simulink model "VEHICLE_DYN_TRAIN"  (R2019b)
settings: Solver=ode4  StartTime=0.0  StopTime=150  FixedStep=0.01  RelTol=1e-3
model workspace (MAT data in the model file):
  ACCEL = [0 0.000975932898663 -0.0414538855996 0.0440661905922 -0.0484817487001 0.0392964510644 -0.0693895143615 0.0261566921783 -0.0586295561215 0.0249771458914 -0.0595081132089 0.0233316013131 ... (544 elements, 17x32)]
  A_mc = 0.000491
  CMD_BR = [0 0 0 0 0 0 0 0 0 0 0 0 ... (15001 elements, 15001x1)]
  CMD_MODE = [1 1 1 1 1 1 1 1 1 1 1 1 ... (15001 elements, 15001x1)]
  CMD_ST = [0 0 0 0 0 0 0 0 0 0 0 0 ... (15001 elements, 15001x1)]
  CMD_T = [0 0.01 0.02 0.03 0.04 0.05 0.06 0.07 0.08 0.09 0.1 0.11 ... (2001 elements, 1x2001)]
  CMD_TH = [0 0 0 0 0 0 0 0 0 0 0 0 ... (15001 elements, 15001x1)]
  CMD_TM = [0 0.01 0.02 0.03 0.04 0.05 0.06 0.07 0.08 0.09 0.1 0.11 ... (15001 elements, 15001x1)]
  CMD_U = [10 10 10 10 10 10 10 10 10 10 10 10 ... (2001 elements, 1x2001)]
  CMD_UX = [0.1 0.1 0.1 0.1 0.1 0.1 0.1 0.1 0.1 0.1 0.1 0.1 ... (15001 elements, 15001x1)]
  COMMAND = [0 0 0 0 0 0 0 0 0 0 0 0 ... (102 elements, 17x6)]
  C_q = 1.4e-06
  DATA_HMMWV : object (value not decoded)
  DATA_VESIM_CC_BRAKE : object (value not decoded)
  FORCE = [0 -4628.45620853 2357.84853747 -1841.82564621 -1727.75397473 1695.19792057 -1263.06335256 1524.31841051 -1649.98396845 -1537.1025145 -1335.96213703 1639.88309903 ... (493 elements, 17x29)]
  F_cf = 80
  F_cs = 138
  F_z = -50097.6
  Gain_v = 70
  J_wheel = 32
  K_vb = 1500
  Kp_rpm = 2.7013
  Kp_v = 30
  L3 = 10
  MIN_TH = 0
  M_sprung = 4672
  M_unsprung = 220
  M_unsprung_front = 220
  M_vehicle = 5112
  N2 = 0
  N3 = 0.01
  P = 36
  P_0 = 10670
  P_gain = 0.0006
  R_wheel = 0.4412
  SLIP = [0 -0.5 0.5 -0.5 -0.5 0.5 -0.5 0.5 -0.5 -0.5 -0.5 0.5 ... (136 elements, 17x8)]
  STATE = [0 4.33747954961e-06 -0.000147430460781 -3.72129119222e-05 -0.000284189368187 -0.000207128204422 -0.00055150808757 -0.000594561033148 -0.000967775941564 -0.00103412952076 -0.00143215770154 -0.00152470872631 ... (544 elements, 17x32)]
  STATES_INIT = [0 0 0.9902452 0 0 1.57079632679 0.01 0 0 0 0 0 ... (32 elements, 1x32)]
  SUSP = [0 -0.00875795294893 -0.00878173856984 -0.00830852863719 -0.00873591176348 -0.00870428588158 -0.00751721170558 -0.00851904716693 -0.00789923296531 -0.00838039895253 -0.00756270047902 -0.00866403364289 ... (612 elements, 17x36)]
  S_o = 3
  T2_r = 4
  TIRE = [0 0.0910654620457 -0.0936729683319 0.0717372732987 0.0513932148365 -0.0365035701266 -0.00739813929507 -0.0045484168787 0.0723881675257 0.0296400174207 -0.0169805208571 0.0207214713062 ... (408 elements, 17x24)]
  TIRELIFTOFF = [0 0 0 0 0 0 0 0 0 0 0 0 ... (17 elements, 17x1)]
  T_LENGTH = 2001
  T_STEP = 0.01
  T_STOP = 12.82
  T_TOTAL = 20
  Ti_rpm = 0.6464
  Ti_v = 2.5
  Tstop = [150 150 150 150 150 150 150 150 150 150 150 150 ... (15001 elements, 15001x1)]
  Tt_rpm = 0.0808
  Tt_v = 0.3125
  U_INIT = 0.01
  b = 170
  brake_Pw = [-3.96235801772 -3.96238075942 -0.895107722214 -0.895547395081 35.9159438465 72.7273668629 152.485661058 244.514654481 330.408495385 364.152342142 462.316700341 535.939857177 ... (40 elements, 40x1)]
  brake_V = [-1.14468402636e-08 6.09303685082e-09 2.9257815427e-07 6.31682445149e-07 8.18779962309e-07 1.05849711081e-06 1.41515318379e-06 1.67826507702e-06 1.8361367918e-06 2.02323385108e-06 2.22788040303e-06 2.46760304614e-06 ... (40 elements, 40x1)]
  diff_efficiency = 0.94
  diff_wRatio = 6.052
  diff_w_ratio = 3.56
  end_time = 140
  engine_inertia = 0.53
  fmin_mg = [42.75 43.31 51.6 64.3 73.65 71.1 72.7 72.36]
  fmin_mg_na = [42.79 42.79 42.79 42.79 42.79 42.79 42.79 42.79]
  g = -9.8
  g_motor_eff = 1
  gr_motor = 0
  i = 5
  mdot_fuel = [5e-06 1e-05 2e-05 3e-05 4e-05 5e-05 6e-05 7e-05 8e-05]
  ms2mph = 2.23694
  n_tire = 4
  no_cyl = 8
  num_points = 14000
  num_points_fast = 140000
  rpm0 = 83.7758040957
  rpm0_c = 1000
  rpm2rads = 0.10471975512
  rpm_e = [50 800 1000 1500 2000 2500 3000 3300]
  rpm_engine = [700 800 1000 1500 2000 2500 3000 3300]
  rpm_hi_idle = 3400
  rpm_idle = 750
  rpm_max_c = 3200
  rpm_rated = 3200
  start_time = 0
  time_step = 0.01
  time_step_fast = 0.001
  torque_engine = [9.767 15.303 12.411 -4.524 -12.214 -35.77 -70 -75.889 75.383 80.318 76.501 61.314 ... (72 elements, 8x9)]
  tout = [0 0.01 0.02 0.03 0.04 0.05 0.06 0.07 0.08 0.09 0.1 0.11 ... (17 elements, 17x1)]
  trq_scale = 0.46
values from neighbouring files (symbols this model uses):
  B = Ref(i:i+2,2)    [Calc_vref.m]    (also in Parameter_load.m = 0.1; VEHICLE_DYN_TRAIN_INIT.m = 0.25)
  Error_now = Error_now_array(end)    [RUN_SIMULATION_SHARED_NEW_POWERTRAIN.m]    (also in VEHICLE_DYN_TRAIN_INIT.m = 0)
  J = 0.075    [VEHICLE_DYN_TRAIN_INIT.m]
  K = 0.075    [VEHICLE_DYN_TRAIN_INIT.m]
  pid2tau_gain = 2.5    [VEHICLE_DYN_TRAIN_INIT.m]
  st_a_in = st_sc_out(end)    [RUN_SIMULATION_SHARED_NEW_POWERTRAIN.m]    (also in VEHICLE_DYN_TRAIN_INIT.m = 0)
  tau_a_in = tau_a_out(end)    [RUN_SIMULATION_SHARED_NEW_POWERTRAIN.m]    (also in VEHICLE_DYN_TRAIN_INIT.m = 0)
undefined symbols (not defined in the file or in its folder): adaptive_flag, autonomy_human_contain_gain, Bias_Distance, dt, error_lookuptable, human_autonomy_agreement_threshold, human_contain_min, human_response_dead_zone, human_torque_max, J_cal, kp_sc, model_lookuptable, Standard_Devices, steering_stable_threshold, UDP_Protocol, vdes, Xobs, Yobs
libraries: simulink x16, sldrtlib x3, dspstat3 x3, vrlib x2
(part 3 of 4)

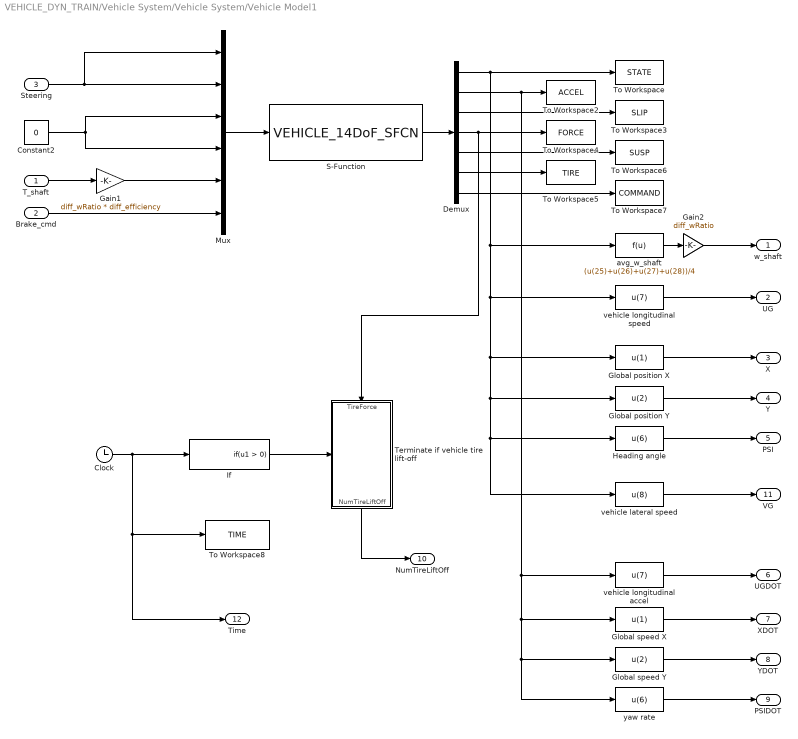
== system VEHICLE_DYN_TRAIN/Vehicle System/Vehicle System/Vehicle Model1 ==
  T_shaft : Inport
  Brake_cmd : Inport  Port=2
  Steering : Inport  Port=3
  Clock : Clock
  Constant2 : Constant  Value=0
  Demux : Demux  Outputs=[32,32,8,29,36,24,6]
  Gain1 : Gain  Gain=diff_wRatio * diff_efficiency
  Gain2 : Gain  Gain=diff_wRatio
  Global position X : Fcn  Expr=u(1)
  Global position Y : Fcn  Expr=u(2)
  Global speed X : Fcn  Expr=u(1)
  Global speed Y : Fcn  Expr=u(2)
  Heading angle : Fcn  Expr=u(6)
  If : If  ShowElse=off
  Mux : Mux  Inputs=6
  S-Function : S-Function  FunctionName=VEHICLE_14DoF_SFCN  SFunctionDeploymentMode=off  EnableBusSupport=off
  Terminate if vehicle tire lift-off : Subsystem  TreatAsAtomicUnit=on
  To Workspace : ToWorkspace  VariableName=STATE  SampleTime=-1
  To Workspace2 : ToWorkspace  VariableName=ACCEL  SampleTime=-1
  To Workspace3 : ToWorkspace  VariableName=SLIP  SampleTime=-1
  To Workspace4 : ToWorkspace  VariableName=FORCE  SampleTime=-1
  To Workspace5 : ToWorkspace  VariableName=TIRE  SampleTime=-1
  To Workspace6 : ToWorkspace  VariableName=SUSP  SampleTime=-1
  To Workspace7 : ToWorkspace  VariableName=COMMAND  SampleTime=-1
  To Workspace8 : ToWorkspace  VariableName=TIME  SampleTime=-1
  avg_w_shaft : Fcn  Expr=(u(25)+u(26)+u(27)+u(28))/4
  vehicle lateral speed : Fcn  Expr=u(8)
  vehicle longitudinal accel : Fcn  Expr=u(7)
  vehicle longitudinal speed : Fcn  Expr=u(7)
  yaw rate : Fcn  Expr=u(6)
  w_shaft : Outport  VectorParamsAs1DForOutWhenUnconnected=off
  UG : Outport  Port=2  VectorParamsAs1DForOutWhenUnconnected=off
  X : Outport  Port=3  VectorParamsAs1DForOutWhenUnconnected=off
  Y : Outport  Port=4  VectorParamsAs1DForOutWhenUnconnected=off
  PSI : Outport  Port=5  VectorParamsAs1DForOutWhenUnconnected=off
  UGDOT : Outport  Port=6  VectorParamsAs1DForOutWhenUnconnected=off
  XDOT : Outport  Port=7  VectorParamsAs1DForOutWhenUnconnected=off
  YDOT : Outport  Port=8  VectorParamsAs1DForOutWhenUnconnected=off
  PSIDOT : Outport  Port=9  VectorParamsAs1DForOutWhenUnconnected=off
  NumTireLiftOff : Outport  Port=10  VectorParamsAs1DForOutWhenUnconnected=off
  VG : Outport  Port=11  VectorParamsAs1DForOutWhenUnconnected=off
  Time : Outport  Port=12  VectorParamsAs1DForOutWhenUnconnected=off
  wires:
  Demux/3 -> To Workspace3/1
  Constant2/1 -> Mux/3, Mux/4
  Demux/5 -> To Workspace6/1
  Steering/1 -> Mux/1, Mux/2
  avg_w_shaft/1 -> Gain2/1
  T_shaft/1 -> Gain1/1
  Demux/7 -> To Workspace7/1
  Demux/1 -> To Workspace/1, vehicle lateral speed/1, Heading angle/1, Global position Y/1, Global position X/1, vehicle longitudinal speed/1, avg_w_shaft/1
  Mux/1 -> S-Function/1
  vehicle longitudinal speed/1 -> UG/1
  Demux/6 -> To Workspace5/1
  Brake_cmd/1 -> Mux/6
  S-Function/1 -> Demux/1
  Heading angle/1 -> PSI/1
  Gain2/1 -> w_shaft/1
  Gain1/1 -> Mux/5
  Global position X/1 -> X/1
  Global position Y/1 -> Y/1
  yaw rate/1 -> PSIDOT/1
  Demux/2 -> vehicle longitudinal accel/1, Global speed X/1, Global speed Y/1, yaw rate/1, To Workspace2/1
  vehicle longitudinal accel/1 -> UGDOT/1
  Global speed X/1 -> XDOT/1
  Global speed Y/1 -> YDOT/1
  Demux/4 -> Terminate if vehicle tire lift-off/1(TireForce), To Workspace4/1
  If/1 -> Terminate if vehicle tire lift-off/Action
  Terminate if vehicle tire lift-off/1(NumTireLiftOff) -> NumTireLiftOff/1
  vehicle lateral speed/1 -> VG/1
  Clock/1 -> Time/1, To Workspace8/1, If/1

== system VEHICLE_DYN_TRAIN/Autonomy/Subsystem/Distance Indicator/Subsystem1 ==
  XG : Inport
  YG : Inport  Port=2
  X_init : Inport  Port=3
  Constant : Constant  Value=0.01
  MATLAB Function : MATLAB Function  TreatAsAtomicUnit=on
  DisInfo : Outport  VectorParamsAs1DForOutWhenUnconnected=off
  X_init_update : Outport  Port=2  VectorParamsAs1DForOutWhenUnconnected=off
  wires:
  X_init/1 -> MATLAB Function/3(Xinit)
  YG/1 -> MATLAB Function/2(Yv)
  XG/1 -> MATLAB Function/1(Xv)
  Constant/1 -> MATLAB Function/4(alpha)
  MATLAB Function/1(Xinit_final) -> X_init_update/1
  MATLAB Function/2(distance) -> DisInfo/1

== system VEHICLE_DYN_TRAIN/Vehicle System/Vehicle System/Powertrain1/DIESEL ENGINE ==
  note: RPM
  note: If you are using MATLAB 6 or earlier,
      | double-click on this look-up table and
      | make sure the "Table data" entry is torque_engine
  engine speed : Inport
  driver  demand : Inport  Port=2
  Engine Map : Lookup2D  RowIndex=rpm_engine  ColumnIndex=mdot_fuel*1e3  Table=torque_engine  SaturateOnIntegerOverflow=on  InputSameDT=on
  Fuel controller/ Governor : Subsystem
  Gain : Gain  Gain=trq_scale  SaturateOnIntegerOverflow=on  OutDataTypeStr=Inherit: Same as input  ParamDataTypeStr=Inherit: Same as input
  Idle Controller : Subsystem
  Mux2 : Mux  Inputs=2
  To File1 : ToFile  Filename=Powertrain_data/engine_NO.mat  MatrixName=engine_out
  radpersec2rpm : Gain  Gain=1/rpm2rads
  engine torque : Outport  VectorParamsAs1DForOutWhenUnconnected=off
  wires:
  radpersec2rpm/1 -> Engine Map/1, Fuel controller/ Governor/2(rpm), Idle Controller/1(engine speed), Mux2/2
  engine speed/1 -> radpersec2rpm/1
  Fuel controller/ Governor/1(mdot_fuel) -> Engine Map/2
  Idle Controller/1(rack) -> Fuel controller/ Governor/1(Rack)
  Gain/1 -> engine torque/1, Mux2/1
  Mux2/1 -> To File1/1
  driver  demand/1 -> Idle Controller/2(driver command)
  Engine Map/1 -> Gain/1

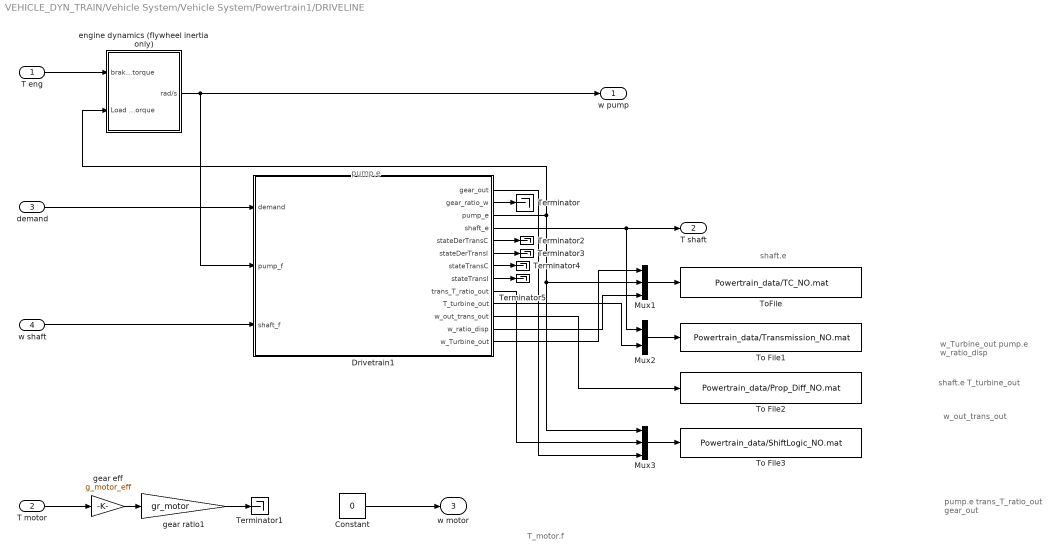
== system VEHICLE_DYN_TRAIN/Vehicle System/Vehicle System/Powertrain1/DRIVELINE ==
  note: pump.e
  note: shaft.e
  note: T_motor.f
  note: w_Turbine_out
      | pump.e
      | w_ratio_disp
  note: shaft.e
      | T_turbine_out
  note: w_out_trans_out
  note: pump.e
      | trans_T_ratio_out
      | gear_out
  "T eng " : Inport
  T motor : Inport  Port=2
  demand : Inport  Port=3
  w shaft : Inport  Port=4
  Constant : Constant  Value=0
  Drivetrain1 : Subsystem  mask(20-sim 4.1 S-Function block){}
      mask help:
      | This block is generated by the 20-sim ANSI-C Code Generator.
      |
      | * look under the mask to get information on the ports
      | * press Help for more detailed information
      | * the parameters of this block are:
      mask Help:
      | This block is generated by the 20-sim ANSI-C Code Generator<br>
      | The block parameters are:<br><blockquote></blockquote>
      | Generated at:<br>
      | <blockquote><b>date:  </b>November 7, 2011<br>
      | <b>time:  </b>6:10:49 pm<br></blockquote>
      | From the following 20-sim model:<br>
      | <blockquote><b>submodel:  </b>Drivetrain<br>
      | <b>model:  </b>model-based internet integration - original drivetrain params<br>
      | <b>file:  </b>C:\Users\Tulga Ersal\Documents\U of M\Post Doc\Projects\Long-haul HIL integration\20-sim\integration models for 20Sim 4.0.1.5 and up\model-based internet integration - original drivetrain params.emx<br>
      | <b>experiment:  </b>C:\Users\Tulga Ersal\Documents\U of M\Post Doc\Projects\Long-haul HIL integration\20-sim\integration models for 20Sim 4.0.1.5 and up\model-based internet integration - original drivetrain params.emx<br></blockquote>
      | Using the following 20-sim license:<br>
      | <blockquote><b>user:  </b>The University of Michigan<br>
      | <b>from:  </b>Student License<br>
      | <b>build: </b>4.1.0.4<br></blockquote>
      mask Display: disp('Drivetrain')
  Mux1 : Mux  Inputs=3
  Mux2 : Mux  Inputs=2
  Mux3 : Mux  Inputs=3
  Terminator{,1..5} (6 alike) : Terminator
  To File1 : ToFile  Filename=Powertrain_data/Transmission_NO.mat  MatrixName=Transmission_out
  To File2 : ToFile  Filename=Powertrain_data/Prop_Diff_NO.mat  MatrixName=Prop_Diff_out
  To File3 : ToFile  Filename=Powertrain_data/ShiftLogic_NO.mat  MatrixName=ShiftLogic_out
  ToFile : ToFile  Filename=Powertrain_data/TC_NO.mat  MatrixName=TC_out
  engine dynamics (flywheel inertia only) : Subsystem
  gear ratio1 : Gain  Gain=gr_motor  SaturateOnIntegerOverflow=on  OutDataTypeStr=Inherit: Same as input  ParamDataTypeStr=Inherit: Same as input
  gear eff : Gain  Gain=g_motor_eff  SaturateOnIntegerOverflow=on  OutDataTypeStr=Inherit: Same as input  ParamDataTypeStr=Inherit: Same as input
  w pump : Outport  InitialOutput=0  VectorParamsAs1DForOutWhenUnconnected=off
  T shaft : Outport  Port=2  InitialOutput=0  VectorParamsAs1DForOutWhenUnconnected=off
  w motor : Outport  Port=3  InitialOutput=0  VectorParamsAs1DForOutWhenUnconnected=off
  wires:
  "T eng "/1 -> engine dynamics (flywheel inertia only)/1(brake torque)
  engine dynamics (flywheel inertia only)/1(rad/s) -> Drivetrain1/2(pump_f), w pump/1
  demand/1 -> Drivetrain1/1(demand)
  w shaft/1 -> Drivetrain1/3(shaft_f)
  T motor/1 -> gear eff/1
  gear eff/1 -> gear ratio1/1
  Constant/1 -> w motor/1
  Mux1/1 -> ToFile/1
  Mux2/1 -> To File1/1
  Mux3/1 -> To File3/1
  gear ratio1/1 -> Terminator1/1
  Drivetrain1/4(shaft_e) -> T shaft/1, Mux2/1
  Drivetrain1/3(pump_e) -> Mux3/1, Mux1/2, engine dynamics (flywheel inertia only)/2(Load Torque)
  Drivetrain1/13(w_Turbine_out) -> Mux1/1
  Drivetrain1/12(w_ratio_disp) -> Mux1/3
  Drivetrain1/10(T_turbine_out) -> Mux2/2
  Drivetrain1/11(w_out_trans_out) -> To File2/1
  Drivetrain1/9(trans_T_ratio_out) -> Mux3/2
  Drivetrain1/1(gear_out) -> Mux3/3
  Drivetrain1/2(gear_ratio_w) -> Terminator/1
  Drivetrain1/5(stateDerTransC) -> Terminator2/1
  Drivetrain1/6(stateDerTransI) -> Terminator3/1
  Drivetrain1/7(stateTransC) -> Terminator4/1
  Drivetrain1/8(stateTransI) -> Terminator5/1

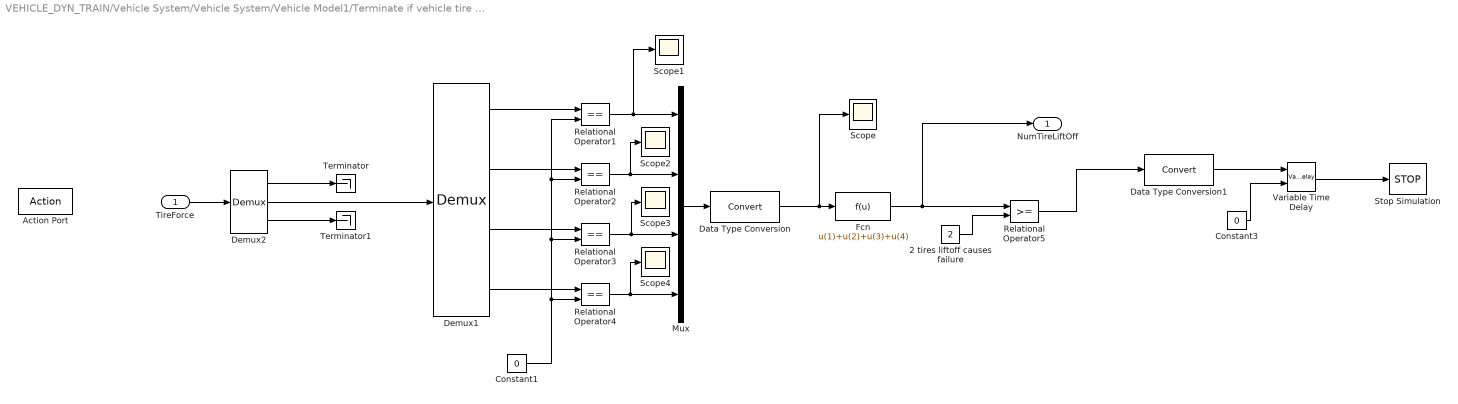
== system VEHICLE_DYN_TRAIN/Vehicle System/Vehicle System/Vehicle Model1/Terminate if vehicle tire lift-off ==
  TireForce : Inport
  Action Port : ActionPort  ActionPortLabel=if(u1 > 0)
  2 tires liftoff causes failure : Constant  Value=2
  Constant1 : Constant  Value=0
  Constant3 : Constant  Value=0
  Data Type Conversion : DataTypeConversion
  Data Type Conversion1 : DataTypeConversion
  Demux1 : Demux
  Demux2 : Demux  Outputs=[8,4,17]
  Fcn : Fcn  Expr=u(1)+u(2)+u(3)+u(4)
  Mux : Mux
  Relational Operator{1..4} (4 alike) : RelationalOperator  Operator===  RndMeth=Nearest  InputSameDT=on
  Relational Operator5 : RelationalOperator  RndMeth=Nearest  InputSameDT=on
  Scope{,1..4} (5 alike) : Scope
  Stop Simulation : Stop
  Terminator : Terminator
  Terminator1 : Terminator
  Variable Time Delay : VariableTransportDelay  MaximumDelay=10  MaximumPoints=10000
  NumTireLiftOff : Outport  InitialOutput=0  VectorParamsAs1DForOutWhenUnconnected=off
  wires:
  Demux2/1 -> Terminator/1
  Demux2/3 -> Terminator1/1
  Demux2/2 -> Demux1/1
  TireForce/1 -> Demux2/1
  Demux1/1 -> Relational Operator1/1
  Demux1/2 -> Relational Operator2/1
  Demux1/3 -> Relational Operator3/1
  Demux1/4 -> Relational Operator4/1
  Relational Operator1/1 -> Scope1/1, Mux/1
  Relational Operator2/1 -> Scope2/1, Mux/2
  Relational Operator3/1 -> Scope3/1, Mux/3
  Relational Operator4/1 -> Scope4/1, Mux/4
  2 tires liftoff causes failure/1 -> Relational Operator5/2
  Mux/1 -> Data Type Conversion/1
  Data Type Conversion/1 -> Scope/1, Fcn/1
  Relational Operator5/1 -> Data Type Conversion1/1
  Constant1/1 -> Relational Operator2/2, Relational Operator1/2, Relational Operator3/2, Relational Operator4/2
  Fcn/1 -> NumTireLiftOff/1, Relational Operator5/1
  Variable Time Delay/1 -> Stop Simulation/1
  Constant3/1 -> Variable Time Delay/2
  Data Type Conversion1/1 -> Variable Time Delay/1

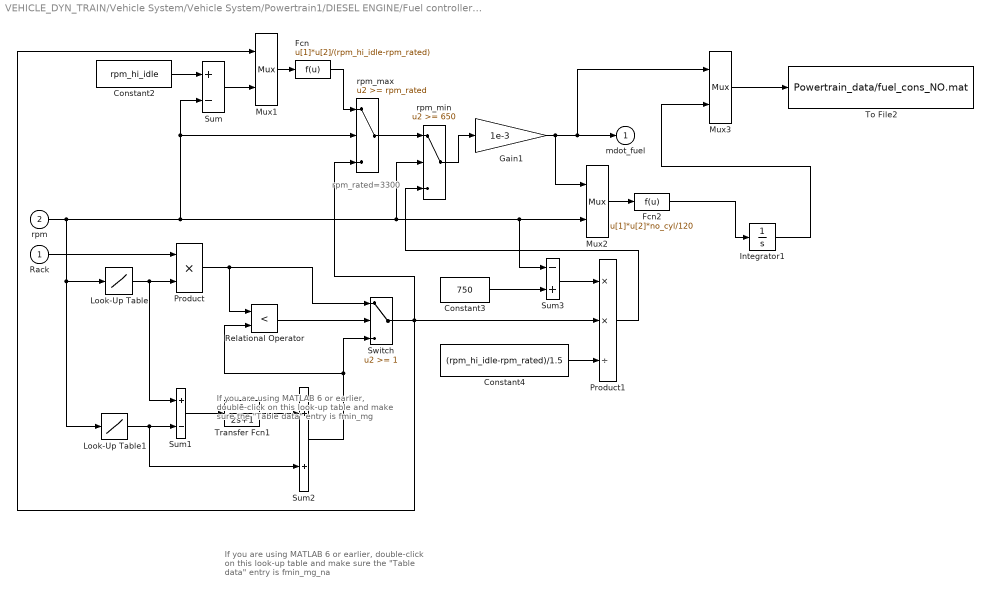
== system VEHICLE_DYN_TRAIN/Vehicle System/Vehicle System/Powertrain1/DIESEL ENGINE/Fuel controller// Governor ==
  note: If you are using MATLAB 6 or earlier,
      | double-click on this look-up table and
      | make sure the "Table data" entry is fmin_mg
  note: If you are using MATLAB 6 or earlier,
      | double-click on this look-up table and
      | make sure the "Table data" entry is fmin_mg_na
  note: rpm_rated=3300
  Rack : Inport
  rpm : Inport  Port=2
  Constant2 : Constant  Value=rpm_hi_idle
  Constant3 : Constant  Value=750
  Constant4 : Constant  Value=(rpm_hi_idle-rpm_rated)/1.5
  Fcn : Fcn  Expr=u[1]*u[2]/(rpm_hi_idle-rpm_rated)
  Fcn2 : Fcn  Expr=u[1]*u[2]*no_cyl/120
  Gain1 : Gain  Gain=1e-3  SaturateOnIntegerOverflow=on  OutDataTypeStr=Inherit: Same as input  ParamDataTypeStr=Inherit: Same as input
  Integrator1 : Integrator
  Look-Up Table : Lookup  InputValues=rpm_e  Table=fmin_mg  SaturateOnIntegerOverflow=on
  Look-Up Table1 : Lookup  InputValues=rpm_e  Table=fmin_mg_na  SaturateOnIntegerOverflow=on
  Mux1 : Mux  Inputs=2
  Mux2 : Mux  Inputs=2
  Mux3 : Mux  Inputs=2
  Product : Product  SaturateOnIntegerOverflow=on  InputSameDT=on  OutDataTypeStr=Inherit: Same as first input
  Product1 : Product  Inputs=**/  SaturateOnIntegerOverflow=on  InputSameDT=on  OutDataTypeStr=Inherit: Same as first input
  Relational Operator : RelationalOperator  Operator=<  RndMeth=Nearest  InputSameDT=on
  Sum : Sum  Inputs=+-  SaturateOnIntegerOverflow=on  InputSameDT=on  OutDataTypeStr=Inherit: Same as first input
  Sum1 : Sum  Inputs=+-  SaturateOnIntegerOverflow=on  InputSameDT=on  OutDataTypeStr=Inherit: Same as first input
  Sum2 : Sum  SaturateOnIntegerOverflow=on  InputSameDT=on  OutDataTypeStr=Inherit: Same as first input
  Sum3 : Sum  Inputs=-+  SaturateOnIntegerOverflow=on  InputSameDT=on  OutDataTypeStr=Inherit: Same as first input
  Switch : Switch  Threshold=1  SaturateOnIntegerOverflow=on  InputSameDT=on
  To File2 : ToFile  Filename=Powertrain_data/fuel_cons_NO.mat  MatrixName=fuel_cons
  Transfer Fcn1 : TransferFcn  Denominator=[2 1]
  rpm_max : Switch  Threshold=rpm_rated  SaturateOnIntegerOverflow=on  InputSameDT=on
  rpm_min : Switch  Threshold=650  SaturateOnIntegerOverflow=on  InputSameDT=on
  mdot_fuel : Outport  InitialOutput=0  VectorParamsAs1DForOutWhenUnconnected=off
  wires:
  Mux3/1 -> To File2/1
  Integrator1/1 -> Mux3/2
  Fcn2/1 -> Integrator1/1
  Switch/1 -> rpm_max/3, Product1/2, Mux1/1
  Product/1 -> Switch/1, Relational Operator/1
  Sum2/1 -> Relational Operator/2, Switch/3
  Relational Operator/1 -> Switch/2
  Look-Up Table1/1 -> Sum2/2, Sum1/2
  Transfer Fcn1/1 -> Sum2/1
  Look-Up Table/1 -> Product/2, Sum1/1
  Sum1/1 -> Transfer Fcn1/1
  Rack/1 -> Product/1
  rpm/1 -> rpm_max/2, Sum/2, Sum3/1, Mux2/2, rpm_min/2, Look-Up Table/1, Look-Up Table1/1
  Fcn/1 -> rpm_max/1
  rpm_max/1 -> rpm_min/1
  Product1/1 -> rpm_min/3
  Constant4/1 -> Product1/3
  Sum3/1 -> Product1/1
  Constant3/1 -> Sum3/2
  Constant2/1 -> Sum/1
  rpm_min/1 -> Gain1/1
  Mux2/1 -> Fcn2/1
  Gain1/1 -> Mux3/1, mdot_fuel/1, Mux2/1
  Sum/1 -> Mux1/2
  Mux1/1 -> Fcn/1

== system VEHICLE_DYN_TRAIN/Vehicle System/Vehicle System/Powertrain1/DIESEL ENGINE/Idle Controller ==
  note: 1/0.6464
  note: 2.7013
  note: 1/(3300-1000)
  note: 750 RPM
  note: anti-windup gain
  note: integral gain
  note: proportional gain
  engine speed : Inport
  driver command : Inport  Port=2
  Gain6 : Gain  Gain=Kp_rpm  SaturateOnIntegerOverflow=on  OutDataTypeStr=Inherit: Same as input  ParamDataTypeStr=Inherit: Same as input
  Gain7 : Gain  Gain=1/Ti_rpm  SaturateOnIntegerOverflow=on  OutDataTypeStr=Inherit: Same as input  ParamDataTypeStr=Inherit: Same as input
  Gain8 : Gain  Gain=1/(rpm_max_c-rpm0_c)  SaturateOnIntegerOverflow=on  OutDataTypeStr=Inherit: Same as input  ParamDataTypeStr=Inherit: Same as input
  Gain9 : Gain  Gain=1/Tt_rpm  SaturateOnIntegerOverflow=on  OutDataTypeStr=Inherit: Same as input  ParamDataTypeStr=Inherit: Same as input
  Idle speed : Constant  Value=rpm_idle
  Integrator2 : Integrator
  Saturation2 : Saturate  UpperLimit=1  LowerLimit=0.005
  Sum5 : Sum  Inputs=-+  SaturateOnIntegerOverflow=on  InputSameDT=on  OutDataTypeStr=Inherit: Same as first input
  Sum6 : Sum  SaturateOnIntegerOverflow=on  InputSameDT=on  OutDataTypeStr=Inherit: Same as first input
  Sum7 : Sum  Inputs=+-  SaturateOnIntegerOverflow=on  InputSameDT=on  OutDataTypeStr=Inherit: Same as first input
  Sum8 : Sum  SaturateOnIntegerOverflow=on  InputSameDT=on  OutDataTypeStr=Inherit: Same as first input
  Switch : Switch  Threshold=.11  SaturateOnIntegerOverflow=on  InputSameDT=on
  rack : Outport  VectorParamsAs1DForOutWhenUnconnected=off
  wires:
  Gain8/1 -> Gain6/1
  Sum7/1 -> Gain8/1
  engine speed/1 -> Sum7/2
  Idle speed/1 -> Sum7/1
  Saturation2/1 -> Sum5/2, rack/1
  driver command/1 -> Switch/2, Switch/1
  Switch/1 -> Sum5/1, Saturation2/1
  Sum6/1 -> Switch/3
  Gain9/1 -> Sum8/2
  Integrator2/1 -> Sum6/2
  Sum8/1 -> Integrator2/1
  Gain7/1 -> Sum8/1
  Sum5/1 -> Gain9/1
  Gain6/1 -> Gain7/1, Sum6/1

== system VEHICLE_DYN_TRAIN/Vehicle System/Vehicle System/Powertrain1/DRIVELINE/Drivetrain1 ==
  demand : Inport
  pump_f : Inport  Port=2
  shaft_f : Inport  Port=3
  Demux : Demux  Outputs=[1 1 1 1 1 1 1 1 1 1 1 1 1 ]
  Mux : Mux  Inputs=[1 1 1 ]
  S-Function : S-Function  FunctionName=Drivetrain  SFunctionDeploymentMode=off  EnableBusSupport=off
  gear_out : Outport  VectorParamsAs1DForOutWhenUnconnected=off
  gear_ratio_w : Outport  Port=2  VectorParamsAs1DForOutWhenUnconnected=off
  pump_e : Outport  Port=3  VectorParamsAs1DForOutWhenUnconnected=off
  shaft_e : Outport  Port=4  VectorParamsAs1DForOutWhenUnconnected=off
  stateDerTransC : Outport  Port=5  VectorParamsAs1DForOutWhenUnconnected=off
  stateDerTransI : Outport  Port=6  VectorParamsAs1DForOutWhenUnconnected=off
  stateTransC : Outport  Port=7  VectorParamsAs1DForOutWhenUnconnected=off
  stateTransI : Outport  Port=8  VectorParamsAs1DForOutWhenUnconnected=off
  trans_T_ratio_out : Outport  Port=9  VectorParamsAs1DForOutWhenUnconnected=off
  T_turbine_out : Outport  Port=10  VectorParamsAs1DForOutWhenUnconnected=off
  w_out_trans_out : Outport  Port=11  VectorParamsAs1DForOutWhenUnconnected=off
  w_ratio_disp : Outport  Port=12  VectorParamsAs1DForOutWhenUnconnected=off
  w_Turbine_out : Outport  Port=13  VectorParamsAs1DForOutWhenUnconnected=off
  wires:
  demand/1 -> Mux/1
  pump_f/1 -> Mux/2
  shaft_f/1 -> Mux/3
  Demux/1 -> gear_out/1
  Demux/2 -> gear_ratio_w/1
  Demux/3 -> pump_e/1
  Demux/4 -> shaft_e/1
  Demux/5 -> stateDerTransC/1
  Demux/6 -> stateDerTransI/1
  Demux/7 -> stateTransC/1
  Demux/8 -> stateTransI/1
  Demux/9 -> trans_T_ratio_out/1
  Demux/10 -> T_turbine_out/1
  Demux/11 -> w_out_trans_out/1
  Demux/12 -> w_ratio_disp/1
  Demux/13 -> w_Turbine_out/1
  Mux/1 -> S-Function/1
  S-Function/1 -> Demux/1

== system VEHICLE_DYN_TRAIN/Vehicle System/Vehicle System/Powertrain1/DRIVELINE/engine dynamics (flywheel inertia only) ==
  brake torque : Inport
  Load Torque : Inport  Port=2
  Engine polar moment of inertia1 : Constant  Value=engine_inertia
  Mux : Mux  Inputs=2
  Sum : Sum  Inputs=+-  SaturateOnIntegerOverflow=on  InputSameDT=on  OutDataTypeStr=Inherit: Same as first input
  calculate omega (replace current init val with value from input file) : Integrator  InitialCondition=0.01*2*pi/60
  div : Fcn  Expr=u[1]/u[2]
  rad/s : Outport  InitialOutput=0  VectorParamsAs1DForOutWhenUnconnected=off
  wires:
  Mux/1 -> div/1
  Sum/1 -> Mux/1
  Load Torque/1 -> Sum/2
  Engine polar moment of inertia1/1 -> Mux/2
  brake torque/1 -> Sum/1
  calculate omega (replace current init val with value from input file)/1 -> rad/s/1
  div/1 -> calculate omega (replace current init val with value from input file)/1

== matlab function VEHICLE_DYN_TRAIN/Autonomy/MATLAB Function ==
  data: u input; y output
function y = fcn(u)

y = u(min(u(104),101));

== matlab function VEHICLE_DYN_TRAIN/MATLAB Function ==
  data: u input; y output; isupdate output
function [y,isupdate]= fcn(u)
   coder.extrinsic('set_param');
   %u: current time; stop time; reference speed; current speed; mode
   y = 0;
   isupdate = 0;
   isupdate = u(6);
   u([3,4])
   if u(5)>0
       % Speed controller
       if u(4) > u(3) && isupdate == 0
           isupdate = 1;
            set_param('VEHICLE_DYN_TRAIN','SimulationCommand','pause')
            disp('Accelerated to reference speed')
       end
   else
       % Varying speed
       if u(1)-u(2)>=-0.005
            set_param('VEHICLE_DYN_TRAIN','SimulationCommand','pause')
            disp('Accelerated to reference speed')
       end
   end

== matlab function VEHICLE_DYN_TRAIN/Autonomy/MATLAB Function4 ==
  data: u input; y output
function y = fcn(u)

y = u(u(104));

== matlab function VEHICLE_DYN_TRAIN/Autonomy/MATLAB Function1 ==
  data: u input; y output
function y = fcn(u)
N = 51;
y = u(N+1);

== matlab function VEHICLE_DYN_TRAIN/Autonomy/MATLAB Function2 ==
  data: u input; y output
function y = fcn(u)

N = 51;
y = u(N+4);

== matlab function VEHICLE_DYN_TRAIN/Haptic Shared Control/Trigger1/MATLAB Function ==
  data: u input; vect output size=[1 10]; vect_old input; tr_vect_old input; threshold input; flag output; tr_vect output size=[1 20]; trigger output
function [vect, flag, tr_vect, trigger] = fcn(u, vect_old, tr_vect_old, threshold)
    vect = zeros(1,10); 
    vect(1,1) = u;
    vect(1,2:10) = vect_old(1:9);
    vect_ordered = sort(vect);
    
    if mean(vect_ordered(1:2)) > threshold
        flag = 1;
    else
        flag = 0;
    end
    
    tr_vect = zeros(1,20);
    tr_vect(1,1) = flag;
    tr_vect(1, 2:20) = tr_vect_old(1:19);
    if sum(tr_vect) == 20
        trigger = 1;
    else
        trigger = 0;
    end
end

== matlab function VEHICLE_DYN_TRAIN/Autonomy/Subsystem/Distance Indicator/Subsystem1/MATLAB Function ==
  data: Xv input; Xinit_final output; Yv input; Xinit input; alpha input; distance output
function [Xinit_final, distance] = DistanceIndicator(Xv, Yv, Xinit, alpha)

    threshold = 0.0005;
    Yinit = 170*sin(0.005*Xinit) + 280*sin(0.001*Xinit) + 50*cos(0.02*Xinit) - 50;
    Yd = 170*0.005*cos(0.005*Xinit) + 280*0.001*cos(0.001*Xinit) - 50*0.02*sin(0.02*Xinit);
    Ydd = -170*0.005*0.005*sin(0.005*Xinit) - 280*0.001*0.001*sin(0.001*Xinit) - 50*0.02*0.02*cos(0.02*Xinit);
    
    Proj = ((Xv - Xinit) + Yd * (Yv - Yinit))/sqrt(1 + Yd^2);
    Projd = (((-1 + Ydd * (Yv - Yinit) - (Yd)^2) * sqrt(1 + Yd^2)) - ((Xv - Xinit + Yd*(Yv - Yinit))) * 1/2 * (1+Yd^2)^(-1/2) * 2 * Yd * Ydd)/(1 + Yd^2);
    
    iter = 1;
    Move = 2 * Proj * Projd;
    
    while (abs(Move * alpha) >= threshold) && (iter <= 1000)
        Xinit = Xinit - alpha * Move;
        Yinit = 170*sin(0.005*Xinit) + 280*sin(0.001*Xinit) + 50*cos(0.02*Xinit) - 50;
        Yd = 170*0.005*cos(0.005*Xinit) + 280*0.001*cos(0.001*Xinit) - 50*0.02*sin(0.02*Xinit);
        Ydd = -170*0.005*0.005*sin(0.005*Xinit) - 280*0.001*0.001*sin(0.001*Xinit) - 50*0.02*0.02*cos(0.02*Xinit);
    
        Proj = ((Xv - Xinit) + Yd * (Yv - Yinit))/sqrt(1 + Yd^2);
        Projd = (((-1 + Ydd * (Yv - Yinit) - (Yd)^2) * sqrt(1 + Yd^2)) - ((Xv - Xinit + Yd*(Yv - Yinit))) * 1/2 * (1+Yd^2)^(-1/2) * 2 * Yd * Ydd)/(1 + Yd^2);
        Move = 2 * Proj * Projd;
        iter = iter + 1;
    end
    
    Xinit_final = Xinit;
    distance = sqrt((Xinit - Xv)^2 + (Yinit - Yv)^2);
end

== matlab function VEHICLE_DYN_TRAIN/Haptic Shared Control/Force Generator/Reference Governor/MATLAB Function ==
  data: ST_C input; ST_RG output; ST_L input
function ST_RG = fcn(ST_C, ST_L)
% ST_d = abs(ST_C - ST_L);
% if ST_d < 0.00075
%     ST_RG = ST_C;
% elseif ST_d < 0.00125
%     ST_RG = ST_L + 0.75*(ST_C - ST_L);
% elseif ST_d < 0.0016
%     ST_RG = ST_L + 0.5*(ST_C - ST_L);
% else
%     ST_RG = ST_L + 0.0016*(ST_C - ST_L)/ST_d;
ST_d = abs(ST_C - ST_L);
ST_diff = ST_C - ST_L;
    if ST_d < 0.0012
        ST_RG = ST_C;
    else
        add_diff = min(ST_d * 0.5, 0.0012) * ST_diff / ST_d;
        ST_RG = ST_L + add_diff;
    end

end

== matlab function VEHICLE_DYN_TRAIN/Vehicle System/MATLAB Function ==
  data: u input; y output
function y = fcn(u)

y = 170*sin(0.005*u)+280*sin(0.001*u)+50*cos(0.02*u)-50;

== matlab function VEHICLE_DYN_TRAIN/Cognitive Workload Estimator/MATLAB Function ==
  data: u input; y output
function y = fcn(u)
if u<45
    y = 0;
elseif u>45 && u<75
    y = 0.5;
else
    y = 0;
end

== matlab function VEHICLE_DYN_TRAIN/Autonomy/MATLAB Function3 ==
  data: flagPrev output; Msg input; iter input; y output; sp output; yOld input; spOld input; t0 input; tStart output; uu output; AS_cnt_Old input; AS_cnt output; Setting input
% function [flagPrev,y, SolFeas,tStart] = fcn(Msg,iter,yOld,SolFeasPrev,t0)
function [flagPrev,y, sp, tStart, uu, AS_cnt] = fcn(Msg,iter,yOld,spOld,t0,AS_cnt_Old,Setting)
% u
% 1-31 st
% 32 comp_time
% 33 cmd_type
% 34 flag
% 35 iter_num
% 36 time_julia
% 37 data ready
% 38 st_hum
% 39 time_simulink

% Input length

tpred = 3;    % s
Npred = 31;     % #
t1 = linspace(0,tpred,Npred);
% Scale to ts = 0.01s
N = 301;
t2 = linspace(0,tpred,N);
uu = interp1(t1,Msg(1:Npred),t2)';
ss = interp1(t1,Msg(Npred+1:2*Npred),t2)';

% Execution window
Nexe = 101;
texe = (Nexe-1)*0.01;
u = [uu(1:Nexe);Msg(2*Npred+1:end)];
s = [ss(1:Nexe);Msg(2*Npred+1:end)];
pred_time = Msg(end-3)/100;

% Current time
t_sml = u(end);

% Initial outputs 
tStart = t0;
flagPrev = 0;
y = yOld;
sp = spOld;
AS_cnt = 0;

% Maximum Hold
MaxHold = 51;  % 0.5s to execute

% Initial case
if iter == 0
    y = u;
    y(1:Nexe) = u(end-1)*ones(Nexe,1);
    sp = s;
    sp(1:Nexe) = s(end-1)*ones(Nexe,1);
    y(Nexe+3) = 1;
    sp(Nexe+3) = 1;
    tStart = t0+0.01;
    return
end

switch Setting
    %% fix update version when optimal solution comes in, active safety
    case 1
        switch u(Nexe+2)
            % NOT OPTIMAL
            case {0,3}
                if yOld(Nexe+2) == 2
                    y = yOld;
                    sp = spOld;

                    y(Nexe+3) = y(Nexe+3)+1;
                    y(end) = u(end);
                    
                    sp(Nexe+3) = sp(Nexe+3)+1;
                    sp(end) = s(end);
                    
                    AS_cnt = AS_cnt_Old +1;
                    
                    if y(Nexe+3) > Nexe
                        y(1:Nexe) = -u(end-1)*ones(Nexe,1);
                        y(Nexe+3) = 1;
                        
                        sp(1:Nexe) = -s(end-1)*ones(Nexe,1);
                        sp(Nexe+3) = 1;
                        
                        AS_cnt = 0;
                        %y(Nexe+2) = 1;  % reset to human mode
                    end
                    
                else
                    y = u;
                    y(1:Nexe) = -u(end-1)*ones(Nexe,1);
                    y(Nexe+3) = 3;
                    
                    sp = s;
                    sp(1:Nexe) = -s(end-1)*ones(Nexe,1);
                    sp(Nexe+3) = 3;
                    
                    AS_cnt = 0;
                end
            % HUMAN FEASIBLE
            case 1
                if yOld(Nexe+2) == 2 && AS_cnt_Old < 10
                    y = yOld;
                    y(Nexe+3) = y(Nexe+3)+1;
                    
                    sp = spOld;
                    sp(Nexe+3) = sp(Nexe+3)+1;
                    
                    if y(Nexe+3) > Nexe
                        y(Nexe+3) = Nexe;
                        sp(Nexe+3) = Nexe;
                    end
                    y(end) = u(end);
                    sp(end) = s(end);
                    AS_cnt = AS_cnt_Old +1;
                else
                    y = u;
                    y(1:Nexe) = -u(end-1)*ones(Nexe,1);
                    
                    sp = s;
                    sp(1:Nexe) = -s(end-1)*ones(Nexe,1);
                    
                    AS_cnt = 0;
                 end
            % HUMAN INFEASIBLE, OPTIMAL
            case 2
                if yOld(Nexe+2) == 1 || yOld(Nexe+2) == 3
                    % Start first solution and execute it
                    AS_cnt = 1;
                    % Copy optimal solution from input
                    y = u;
                    sp = s;
                    t_julia = u(end-3);     
                    delay = t_sml - t_julia;
                    flagPrev = floor(delay/0.01)+2;
                    % Chop off signals
                    y(1:Nexe) = uu(flagPrev:(flagPrev+100));
                    sp(1:Nexe) = ss(flagPrev:(flagPrev+100));
                    % Shift the signals
                    y(1:Nexe) = y(1:Nexe) - (y(1)- (-u(end-1)) );
                    sp(1:Nexe) = sp(1:Nexe) - (sp(1)- (-s(end-1)) );
                %% Still in optimal solution
                else
                    % no new message
                    if u(end-2) == 0
                        y = yOld;
                        y(Nexe+3) = y(Nexe+3)+1;
                        
                        sp = spOld;
                        sp(Nexe+3) = sp(Nexe+3)+1;
                        
                        if y(Nexe+3) > Nexe
                            y(Nexe+3) = Nexe;
                            sp(Nexe+3) = Nexe;
                        end
                        y(end) = u(end);
                        sp(end) = s(end);
                        AS_cnt = AS_cnt_Old +1;
                        if AS_cnt_Old > MaxHold
                            AS_cnt = 1;
                        end
                    % new message, create a buffer
                    else
                        if AS_cnt_Old >= 10 || yOld(Nexe+4) == 1  % 1
                            AS_cnt = 1;
                            % Copy optimal solution from input
                            y = u;
                            sp = s;
                            t_julia = u(end-3);     
                            delay = t_sml - t_julia;
                            flagPrev = floor(delay/0.01)+2;
                            if flagPrev >= Nexe
                                flagPrev = Nexe;
                            end
                            % Chop off signals
                            y(1:Nexe) = uu(flagPrev:flagPrev+100);
                            % Shift the signals
                            y(1:Nexe) = y(1:Nexe) - (y(1)- yOld(yOld(Nexe+3)+1) );
                            
                            sp(1:Nexe) = ss(flagPrev:flagPrev+100);
                            % Shift the signals
                            sp(1:Nexe) = sp(1:Nexe) - (sp(1)- spOld(spOld(Nexe+3)+1) );
                        else
                            y = yOld;
                            y(Nexe+3) = y(Nexe+3)+1;
                            
                            sp = spOld;
                            sp(Nexe+3) = sp(Nexe+3)+1;
                            
                            if y(Nexe+3) > Nexe
                                y(Nexe+3) = Nexe;
                                sp(Nexe+3) = Nexe;
                            end
                            y(end) = u(end);
                            sp(end) = s(end);
                            AS_cnt = AS_cnt_Old +1;
                        end
                    end
                end
                
        end
      
    %% varying update version, haptic shared control    
    case {0,2,4}
%         if u(Nexe+2) == 3
%             if yOld(Nexe+2) == 2
%                 y = yOld;
%                 y(Nexe+3) = y(Nexe+3)+1;
%                 y(end) = u(end);
%                 
%                 sp = spOld;
%                 sp(Nexe+3) = sp(Nexe+3)+1;
%                 sp(end) = s(end);
% 
%                 if y(Nexe+3) > Nexe
%                     y(1:Nexe) = u(Nexe)*ones(Nexe,1);
%                     y(Nexe+3) = 1;
%                     
%                     sp(1:Nexe) = s(Nexe)*ones(Nexe,1);
%                     sp(Nexe+3) = 1;
%                     
%                     AS_cnt = 0;
%                    % y(Nexe+2) = 1;  % reset to human mode
%                 end        
%             else
%                 y = u;
%                 y(1:Nexe) = u(Nexe)*ones(Nexe,1);
%                 y(Nexe+3) = 1;
%                 
%                 sp = s;
%                 sp(1:Nexe) = s(Nexe)*ones(Nexe,1);
%                 sp(Nexe+3) = 1;
%             end
%             
%         else
            if u(end-5) > 0 
                y = u;  
                sp = s;  
                if u(Nexe+4) > 1
                    t_julia = u(end-4);     % time when vehicle is at, 7.21s, #38
                    delay = t_sml - t_julia;    % delay in vehicle state, 7.33-7.21
                    delay = delay - pred_time;
                    if delay < 0
                        delay = 0;
                    end
                    flagPrev = floor(delay/0.01)+1;
                    if flagPrev >=  Nexe
                        flagPrev = Nexe;
                    end
                else
                    flagPrev = 1;
                end
                % Chop off signals
                y(1:Nexe) = uu(flagPrev:(flagPrev+100));
                sp(1:Nexe) = ss(flagPrev:(flagPrev+100));
                % Shift the signals
%                 if yOld(Nexe+2) == 2
%                     y(1:Nexe) = y(1:Nexe) - (y(1)- yOld(yOld(Nexe+3)+1) );
%                 else
%                     y(1:Nexe) = y(1:Nexe) - (y(1)- (-u(end-1)) );
%                 end
                y(Nexe+3) = 1;
                sp(Nexe+3) = 1;
                
                % fight exists and automation complies
%                 if abs(y(1)- (-u(end-1)) ) >= 0.025   % 0.03
%                     y(1:Nexe) = -u(end-1)*ones(Nexe,1);
% %                    y(Nexe+2) = 1;
%                 end

            else
                % Continue previous solution
%                 if yOld(Nexe+2) == 2
                    y = yOld;
                    sp = spOld;
                    % Increase flag
                    y(Nexe+3) = y(Nexe+3)+1;
                    
                    sp(Nexe+3) = sp(Nexe+3)+1;
                    
                    if y(Nexe+3) > Nexe
                        y(Nexe+3) = Nexe;
                        y(end-1) = u(end-1);
                        
                        sp(Nexe+3) = Nexe;
                        sp(end-1) = s(end-1);
                    end
                    y(end) = u(end);
                    sp(end) = s(end);
                % Use human command
%                 else
%                     y = yOld;
%                     y(1:Nexe) = u(end-1)*ones(Nexe,1);
%                     y(Nexe+3) = y(Nexe+3)+1;
%                     if y(Nexe+3) > Nexe
%                         y(Nexe+3) = Nexe;
%                         y(end-1) = u(end-1);
%                     end
%                     y(end) = u(end);
%                 end
            end
%         end
    
    %% teleoperation
    case 3
        y = u;
        y(1:Nexe) = -u(end-1)*ones(Nexe,1);
        y(Nexe+3) = 1;
        
        sp = s;
        sp(1:Nexe) = -s(end-1)*ones(Nexe,1);
        sp(Nexe+3) = 1;
              
        
        
        
    %% fixed update version  
    case 5
        % Update every texe
        if mod(t_sml-tStart+0.01,texe) >= texe || mod(t_sml-tStart+0.01,texe) < 0.01  
            % Find the latest feasible solution if the current one is
            % infeasible ,need ++++ 
%             if u(Nexe+2) == 3
%                 u = SolFeasPrev;
%             end
            t_julia = u(end-3);     % time when vehicle is at, 7.32s
            y = u; % new input, #39
            sp = s;
            
            if u(Nexe+4) > 1   % need prediction
                delay = t_sml - t_julia;    % delay in vehicle state, 7.69-7.32
                flagPrev = floor(delay/0.01)+1;    
            else
                flagPrev = 1;
            end
            if flagPrev >=  Nexe
                flagPrev = Nexe;
            end

            % prediction
            y(1:Nexe) = uu(flagPrev:(flagPrev+100));
            sp(1:Nexe) = ss(flagPrev:(flagPrev+100));
            disp('Predict')
        else
            y = yOld;
            sp = spOld;
            % Increase flag
            y(Nexe+3) = y(Nexe+3)+1;
            sp(Nexe+3) = sp(Nexe+3)+1;
            if y(Nexe+3) > Nexe
                y(Nexe+3) = Nexe;
                y(end-1) = u(end-1);
                sp(Nexe+3) = Nexe;
                sp(end-1) = s(end-1);
            end
            y(end) = u(end);
            sp(end) = s(end);
        end
        
end
                    
end

== matlab function VEHICLE_DYN_TRAIN/Autonomy/Subsystem/Subsystem/MATLAB Function ==
  data: XG input; Xobs_pass output; Yobs_pass output; YG input; PHIG input; Xobs input; Yobs input; vdes input
function [Xobs_pass,Yobs_pass] = fcn(XG,YG,PHIG,Xobs,Yobs,vdes)
    Xobs_seen = Xobs(1:8);
    Yobs_seen = Yobs(1:8);
    N = length(Xobs_seen);
    Xveh = XG*ones(N,1);
    Yveh = YG*ones(N,1);
    ObsR = 1*ones(N,1);
    sm = 2;
    Dist = sqrt( (Xveh-Xobs_seen).^2+(Yveh-Yobs_seen).^2 );
    Dir = atan2(Yobs_seen-Yveh, Xobs_seen-Xveh );
    % find front and out of safe margin, else 0
    ActiveAll = double(abs(Dir-PHIG)<=pi/2 & Dist>=ObsR+sm & Dist <=10*vdes );    
    
    Dist = Dist.* ActiveAll;
    for i = 1:length(Dist)
        if Dist(i) == 0
            Dist(i) = 2000;
        end
    end
    [Distsort,sortIdx] = sort(Dist);
    InvalidAll = double(Distsort == 2000);
    
    % Obstacles in the front 
    Xobs_inview = Xobs(sortIdx)+InvalidAll*900;
    Yobs_inview = Yobs(sortIdx)+InvalidAll*900;
    
    Xobs_pass = Xobs_inview(1:3);
    Yobs_pass = Yobs_inview(1:3);

== matlab function VEHICLE_DYN_TRAIN/Autonomy/MATLAB Function5 ==
  data: u input; y output
function y = fcn(u)

y = u(min(u(104),101));
